simulink model "gm_transmitter"  (R2020b)
settings: Solver=FixedStepDiscrete  StartTime=0.0  StopTime=100000  RelTol=1e-3
undefined symbols (not defined in the file or in its folder): message
libraries: hdlmdlgenlib x98, dspsigops x53, hdlsllib x22, simulink x11, dspmlti4 x2, whdlio x1
(part 2 of 3)

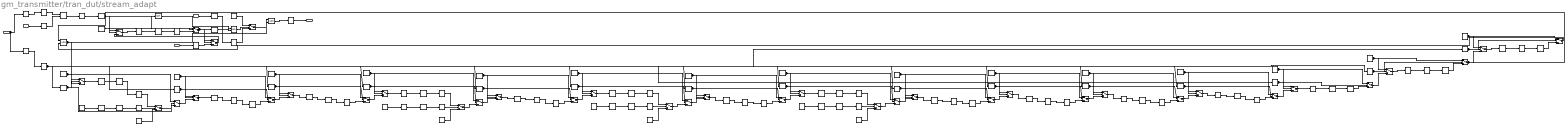
== system gm_transmitter/tran_dut/stream_adapt ==
  note: Padding unit
  input_bit : Inport  OutDataTypeStr=fixdt(0, 1, 0)  PortDimensions=1  SampleTime=2.06577425218972
  start : Inport  Port=2  OutDataTypeStr=boolean  PortDimensions=1  SampleTime=0.258221781523715
  valid : Inport  Port=3  OutDataTypeStr=boolean  PortDimensions=1  SampleTime=2.06577425218972
  end : Inport  Port=4  OutDataTypeStr=boolean  PortDimensions=1  SampleTime=0.258221781523715
  Compare To Constant : simulink/Logic and Bit Operations/Compare To Constant  relop=>=  const="fi(0,0,16,0,\"hex\",\"bd18\")"  OutDataTypeStr=boolean
  Compare To Constant1 : simulink/Logic and Bit Operations/Compare To Constant  relop===  const="fi(0,0,1,0,\"hex\",\"1\")"  OutDataTypeStr=boolean
  Constant : Constant  Value=0  OutDataTypeStr=fixdt(0, 1, 1000)  SampleTime=0.258221781523715
  Delay10_lowered : RateTransition  OutPortSampleTimeOpt=Multiple of input port sample time  OutPortSampleTimeMultiple=8
  Delay11_lowered : RateTransition  OutPortSampleTimeOpt=Multiple of input port sample time  OutPortSampleTimeMultiple=8
  Delay12_lowered : RateTransition  OutPortSampleTimeOpt=Multiple of input port sample time  OutPortSampleTimeMultiple=8
  Delay13_lowered : RateTransition  OutPortSampleTimeOpt=Multiple of input port sample time  OutPortSampleTimeMultiple=8
  Delay14_lowered : RateTransition  OutPortSampleTimeOpt=Multiple of input port sample time  OutPortSampleTimeMultiple=8
  Delay1_lowered : RateTransition  OutPortSampleTimeOpt=Multiple of input port sample time  OutPortSampleTimeMultiple=8
  Delay2_lowered : RateTransition  OutPortSampleTimeOpt=Multiple of input port sample time  OutPortSampleTimeMultiple=8
  Delay3_lowered : RateTransition  OutPortSampleTimeOpt=Multiple of input port sample time  OutPortSampleTimeMultiple=8
  Delay3_lowered_Initial_Val : Constant  OutDataTypeStr=boolean  SampleTime=0.258221781523715
  Delay3_lowered_ctrl_const : Constant  OutDataTypeStr=boolean  SampleTime=2.06577425218972
  Delay3_lowered_switch : Switch  Criteria=u2 ~= 0  Threshold=double(0)  OutDataTypeStr=boolean  SampleTime=0.258221781523715
  Delay4_lowered : RateTransition  OutPortSampleTimeOpt=Multiple of input port sample time  OutPortSampleTimeMultiple=8
  Delay5_lowered : RateTransition  OutPortSampleTimeOpt=Multiple of input port sample time  OutPortSampleTimeMultiple=8
  Delay5_lowered_Initial_Val : Constant  OutDataTypeStr=boolean  SampleTime=0.258221781523715
  Delay5_lowered_ctrl_const : Constant  OutDataTypeStr=boolean  SampleTime=2.06577425218972
  Delay5_lowered_switch : Switch  Criteria=u2 ~= 0  Threshold=double(0)  OutDataTypeStr=boolean  SampleTime=0.258221781523715
  Delay6_lowered : RateTransition  OutPortSampleTimeOpt=Multiple of input port sample time  OutPortSampleTimeMultiple=8
  Delay7_lowered : RateTransition  OutPortSampleTimeOpt=Multiple of input port sample time  OutPortSampleTimeMultiple=8
  Delay7_lowered_Initial_Val : Constant  OutDataTypeStr=boolean  SampleTime=0.258221781523715
  Delay7_lowered_ctrl_const : Constant  OutDataTypeStr=boolean  SampleTime=2.06577425218972
  Delay7_lowered_switch : Switch  Criteria=u2 ~= 0  Threshold=double(0)  OutDataTypeStr=boolean  SampleTime=0.258221781523715
  Delay8_lowered : RateTransition  OutPortSampleTimeOpt=Multiple of input port sample time  OutPortSampleTimeMultiple=8
  Delay9_lowered : RateTransition  OutPortSampleTimeOpt=Multiple of input port sample time  OutPortSampleTimeMultiple=8
  Delay_lowered : RateTransition  OutPortSampleTimeOpt=Multiple of input port sample time  OutPortSampleTimeMultiple=8
  Delay_lowered_Initial_Val : Constant  OutDataTypeStr=boolean  SampleTime=0.258221781523715
  Delay_lowered_ctrl_const : Constant  OutDataTypeStr=boolean  SampleTime=2.06577425218972
  Delay_lowered_switch : Switch  Criteria=u2 ~= 0  Threshold=double(0)  OutDataTypeStr=boolean  SampleTime=0.258221781523715
  From{,1..14} (15 alike) : hdlmdlgenlib/Buffer
      settings: SourceProductBaseCode=SL
  Goto : hdlmdlgenlib/Buffer
      settings: SourceProductBaseCode=SL
  Initial_Val{,1..7,9,11,13..14} (12 alike) : Constant  Value=0  OutDataTypeStr=boolean  SampleTime=0.258221781523715
  Initial_Val{8,10,12,15} (4 alike) : Constant  OutDataTypeStr=boolean  SampleTime=0.258221781523715
  Logical Operator : Logic  Operator=XOR  AllPortsSameDT=off  OutDataTypeStr=boolean  SampleTime=0.258221781523715
  Logical Operator1 : Logic  Operator=XOR  AllPortsSameDT=off  OutDataTypeStr=boolean  SampleTime=0.258221781523715
  Logical Operator2 : Logic  Operator=NOT  Inputs=1  AllPortsSameDT=off  OutDataTypeStr=boolean  SampleTime=0.258221781523715
  Logical Operator3 : Logic  AllPortsSameDT=off  OutDataTypeStr=boolean  SampleTime=0.258221781523715
  RateTransition : RateTransition  OutPortSampleTimeOpt=Multiple of input port sample time  OutPortSampleTimeMultiple=8
  Switch : Switch  Criteria=u2 ~= 0  Threshold=double(0)  OutDataTypeStr=boolean  SampleTime=0.258221781523715
  Switch1 : Switch  Criteria=u2 ~= 0  Threshold=double(0)  OutDataTypeStr=fixdt(0, 1, 0)  SampleTime=0.258221781523715
  crp_delay : Delay  DelayLength=double(1)  InitialCondition=0  SampleTime=0.258221781523715
  crp_out_delay{,1..15} (16 alike) : Delay  DelayLength=double(1)  InitialCondition=0  SampleTime=0.258221781523715
  delayMatch{,1..3,5,8..12} (10 alike) : Delay  DelayLength=double(1)  InitialCondition=0  SampleTime=2.06577425218972
  delayMatch4 : Delay  DelayLength=double(1)  InitialCondition=0  SampleTime=0.258221781523715
  delayMatch6 : Delay  DelayLength=double(8)  InitialCondition=0  SampleTime=0.258221781523715
  delayMatch7 : Delay  DelayLength=double(8)  InitialCondition=0  SampleTime=0.258221781523715
  ended_flag_lowered : RateTransition  OutPortSampleTimeOpt=Multiple of input port sample time  OutPortSampleTimeMultiple=8
  frame_counter : hdlsllib/Sources/HDL Counter  CountType=Count limited  CountInit=double(0)  CountStep=double(1)  CountMax=double(48408)  CountFromType=Initial value  CountFrom=double(0)  CountResetPort=on  CountLoadPort=off  CountEnbPort=on  CountDirPort=off  CountDataType=Unsigned  CountWordLen=16  CountFracLen=0  CountSampTime=2.06577425218972
  in10_repeat : dspsigops/Repeat  N=double(8)  RateOptions=Allow multirate processing  ic=0  mode=Unused parameter value
  in11_repeat : dspsigops/Repeat  N=double(8)  RateOptions=Allow multirate processing  ic=0  mode=Unused parameter value
  in12_repeat : dspsigops/Repeat  N=double(8)  RateOptions=Allow multirate processing  ic=0  mode=Unused parameter value
  in13_repeat : dspsigops/Repeat  N=double(8)  RateOptions=Allow multirate processing  ic=0  mode=Unused parameter value
  in14_repeat : dspsigops/Repeat  N=double(8)  RateOptions=Allow multirate processing  ic=0  mode=Unused parameter value
  in15_repeat : dspsigops/Repeat  N=double(8)  RateOptions=Allow multirate processing  ic=0  mode=Unused parameter value
  in16_repeat : dspsigops/Repeat  N=double(8)  RateOptions=Allow multirate processing  ic=0  mode=Unused parameter value
  in17_repeat : dspsigops/Repeat  N=double(8)  RateOptions=Allow multirate processing  ic=0  mode=Unused parameter value
  in18_repeat : dspsigops/Repeat  N=double(8)  RateOptions=Allow multirate processing  ic=0  mode=Unused parameter value
  in19_repeat : dspsigops/Repeat  N=double(8)  RateOptions=Allow multirate processing  ic=0  mode=Unused parameter value
  in20_repeat : dspsigops/Repeat  N=double(8)  RateOptions=Allow multirate processing  ic=0  mode=Unused parameter value
  in21_repeat : dspsigops/Repeat  N=double(8)  RateOptions=Allow multirate processing  ic=0  mode=Unused parameter value
  in22_repeat : dspsigops/Repeat  N=double(8)  RateOptions=Allow multirate processing  ic=0  mode=Unused parameter value
  in23_repeat : dspsigops/Repeat  N=double(8)  RateOptions=Allow multirate processing  ic=0  mode=Unused parameter value
  in2_repeat : dspsigops/Repeat  N=double(8)  RateOptions=Allow multirate processing  ic=0  mode=Unused parameter value
  in3_repeat : dspsigops/Repeat  N=double(8)  RateOptions=Allow multirate processing  ic=0  mode=Unused parameter value
  in4_repeat : dspsigops/Repeat  N=double(8)  RateOptions=Allow multirate processing  ic=0  mode=Unused parameter value
  in5_repeat : dspsigops/Repeat  N=double(8)  RateOptions=Allow multirate processing  ic=0  mode=Unused parameter value
  in6_repeat : dspsigops/Repeat  N=double(8)  RateOptions=Allow multirate processing  ic=0  mode=Unused parameter value
  in7_repeat : dspsigops/Repeat  N=double(8)  RateOptions=Allow multirate processing  ic=0  mode=Unused parameter value
  in8_repeat : dspsigops/Repeat  N=double(8)  RateOptions=Allow multirate processing  ic=0  mode=Unused parameter value
  in9_repeat : dspsigops/Repeat  N=double(8)  RateOptions=Allow multirate processing  ic=0  mode=Unused parameter value
  reset_in{,1..15} (16 alike) : Switch  Criteria=u2 ~= 0  Threshold=double(0)  OutDataTypeStr=boolean  SampleTime=0.258221781523715
  reset_out{,1..15} (16 alike) : Switch  Criteria=u2 ~= 0  Threshold=double(0)  OutDataTypeStr=boolean  SampleTime=0.258221781523715
  out : Outport  VectorParamsAs1DForOutWhenUnconnected=off
  wires:
  frame_counter/1 -> in23_repeat/1
  delayMatch11/1 -> in20_repeat/1
  delayMatch10/1 -> in16_repeat/1
  delayMatch9/1 -> in13_repeat/1
  delayMatch8/1 -> in10_repeat/1
  delayMatch12/1 -> in21_repeat/1
  delayMatch7/1 -> Goto/1
  delayMatch5/1 -> frame_counter/2
  delayMatch6/1 -> Switch/3
  crp_delay/1 -> RateTransition/1
  RateTransition/1 -> frame_counter/1
  input_bit/1 -> delayMatch12/1
  start/1 -> delayMatch7/1, crp_delay/1
  valid/1 -> delayMatch5/1
  end/1 -> delayMatch6/1
  delayMatch3/1 -> delayMatch8/1
  delayMatch2/1 -> delayMatch9/1
  delayMatch1/1 -> delayMatch10/1
  delayMatch/1 -> delayMatch11/1
  ended_flag_lowered/1 -> in22_repeat/1
  Delay_lowered/1 -> in19_repeat/1
  Delay1_lowered/1 -> in18_repeat/1
  Delay2_lowered/1 -> in17_repeat/1
  Delay3_lowered/1 -> in15_repeat/1
  Delay4_lowered/1 -> in14_repeat/1
  Delay5_lowered/1 -> in12_repeat/1
  Delay6_lowered/1 -> in11_repeat/1
  Delay7_lowered/1 -> in9_repeat/1
  Delay8_lowered/1 -> in8_repeat/1
  Delay9_lowered/1 -> in7_repeat/1
  Delay10_lowered/1 -> in6_repeat/1
  Delay11_lowered/1 -> in5_repeat/1
  Delay12_lowered/1 -> in4_repeat/1
  Delay13_lowered/1 -> in3_repeat/1
  Delay14_lowered/1 -> in2_repeat/1
  Delay_lowered_ctrl_const/1 -> delayMatch/1
  Delay3_lowered_ctrl_const/1 -> delayMatch1/1
  Delay5_lowered_ctrl_const/1 -> delayMatch2/1
  Delay7_lowered_ctrl_const/1 -> delayMatch3/1
  crp_out_delay/1 -> ended_flag_lowered/1
  crp_out_delay1/1 -> Delay_lowered/1
  crp_out_delay2/1 -> Delay1_lowered/1
  crp_out_delay3/1 -> Delay2_lowered/1
  crp_out_delay4/1 -> Delay3_lowered/1
  crp_out_delay5/1 -> Delay4_lowered/1
  crp_out_delay6/1 -> Delay5_lowered/1
  crp_out_delay7/1 -> Delay6_lowered/1
  crp_out_delay8/1 -> Delay7_lowered/1
  crp_out_delay9/1 -> Delay8_lowered/1
  crp_out_delay10/1 -> Delay9_lowered/1
  crp_out_delay11/1 -> Delay10_lowered/1
  crp_out_delay12/1 -> Delay11_lowered/1
  crp_out_delay13/1 -> Delay12_lowered/1
  crp_out_delay14/1 -> Delay13_lowered/1
  crp_out_delay15/1 -> Delay14_lowered/1
  in2_repeat/1 -> reset_out/3
  in3_repeat/1 -> reset_out1/3
  in4_repeat/1 -> reset_out2/3
  in5_repeat/1 -> reset_out3/3
  in6_repeat/1 -> reset_out4/3
  in7_repeat/1 -> reset_out5/3
  in8_repeat/1 -> reset_out6/3
  in9_repeat/1 -> Delay7_lowered_switch/1
  in10_repeat/1 -> Delay7_lowered_switch/2
  in11_repeat/1 -> reset_out8/3
  in12_repeat/1 -> Delay5_lowered_switch/1
  in13_repeat/1 -> Delay5_lowered_switch/2
  in14_repeat/1 -> reset_out10/3
  in15_repeat/1 -> Delay3_lowered_switch/1
  in16_repeat/1 -> Delay3_lowered_switch/2
  in17_repeat/1 -> reset_out12/3
  in18_repeat/1 -> reset_out13/3
  in19_repeat/1 -> Delay_lowered_switch/1
  in20_repeat/1 -> Delay_lowered_switch/2
  in21_repeat/1 -> Switch1/3
  in22_repeat/1 -> reset_out15/3
  in23_repeat/1 -> Compare To Constant/1
  delayMatch4/1 -> out/1
  Initial_Val/1 -> reset_out15/1, reset_in/1
  Switch/1 -> reset_in/3
  From9/1 -> reset_out5/2, reset_in6/2
  From8/1 -> reset_out6/2, reset_in7/2
  From7/1 -> reset_out7/2, reset_in8/2
  From6/1 -> reset_out8/2, reset_in9/2
  From5/1 -> reset_out9/2, reset_in10/2
  From4/1 -> reset_out10/2, reset_in11/2
  From3/1 -> reset_out11/2, reset_in12/2
  From2/1 -> reset_out12/2, reset_in13/2
  From13/1 -> reset_out1/2, reset_in2/2
  From12/1 -> reset_out2/2, reset_in3/2
  From11/1 -> reset_out3/2, reset_in4/2
  From10/1 -> reset_out4/2, reset_in5/2
  From1/1 -> reset_out13/2, reset_in14/2
  From/1 -> reset_out14/2, reset_in15/2
  Goto/1 -> From9/1, From8/1, From7/1, From6/1, From5/1, From4/1, From3/1, From2/1, From14/1, From13/1, From12/1, From11/1, From10/1, From1/1, From/1
  From14/1 -> reset_out/2, reset_in1/2
  reset_out/1 -> Logical Operator/2
  Initial_Val1/1 -> reset_out/1, reset_in1/1
  reset_out1/1 -> Logical Operator/1, reset_in1/3
  Initial_Val2/1 -> reset_out1/1, reset_in2/1
  reset_out2/1 -> reset_in2/3
  Initial_Val3/1 -> reset_out2/1, reset_in3/1
  reset_out3/1 -> reset_in3/3
  Initial_Val4/1 -> reset_out3/1, reset_in4/1
  reset_out4/1 -> reset_in4/3
  Initial_Val5/1 -> reset_out4/1, reset_in5/1
  reset_out5/1 -> reset_in5/3
  Initial_Val6/1 -> reset_out5/1, reset_in6/1
  reset_out6/1 -> reset_in6/3
  Initial_Val7/1 -> reset_out6/1, reset_in7/1
  Delay7_lowered_Initial_Val/1 -> Delay7_lowered_switch/3
  Delay7_lowered_switch/1 -> reset_out7/3
  reset_out7/1 -> reset_in7/3
  Initial_Val8/1 -> reset_out7/1, reset_in8/1
  reset_out8/1 -> reset_in8/3
  Initial_Val9/1 -> reset_out8/1, reset_in9/1
  Delay5_lowered_Initial_Val/1 -> Delay5_lowered_switch/3
  Delay5_lowered_switch/1 -> reset_out9/3
  reset_out9/1 -> reset_in9/3
  Initial_Val10/1 -> reset_out9/1, reset_in10/1
  reset_out10/1 -> reset_in10/3
  Initial_Val11/1 -> reset_out10/1, reset_in11/1
  Delay3_lowered_Initial_Val/1 -> Delay3_lowered_switch/3
  Delay3_lowered_switch/1 -> reset_out11/3
  reset_out11/1 -> reset_in11/3
  Initial_Val12/1 -> reset_out11/1, reset_in12/1
  reset_out12/1 -> reset_in12/3
  Initial_Val13/1 -> reset_out12/1, reset_in13/1
  reset_out13/1 -> reset_in13/3
  Initial_Val14/1 -> reset_out13/1, reset_in14/1
  Delay_lowered_Initial_Val/1 -> Delay_lowered_switch/3
  Delay_lowered_switch/1 -> reset_out14/3
  reset_out14/1 -> reset_in14/3
  Initial_Val15/1 -> reset_out14/1, reset_in15/1
  Logical Operator/1 -> Logical Operator1/1, reset_in15/3
  Constant/1 -> Switch1/1
  Switch1/1 -> Logical Operator1/2
  Logical Operator2/1 -> Logical Operator3/1
  Logical Operator3/1 -> Switch1/2
  Compare To Constant1/1 -> Logical Operator3/2
  reset_out15/1 -> Compare To Constant1/1, Switch/2, Switch/1
  Compare To Constant/1 -> Logical Operator2/1, reset_out15/2, reset_in/2
  reset_in/1 -> crp_out_delay/1
  reset_in15/1 -> crp_out_delay1/1
  reset_in14/1 -> crp_out_delay2/1
  reset_in13/1 -> crp_out_delay3/1
  reset_in12/1 -> crp_out_delay4/1
  reset_in11/1 -> crp_out_delay5/1
  reset_in10/1 -> crp_out_delay6/1
  reset_in9/1 -> crp_out_delay7/1
  reset_in8/1 -> crp_out_delay8/1
  reset_in7/1 -> crp_out_delay9/1
  reset_in6/1 -> crp_out_delay10/1
  reset_in5/1 -> crp_out_delay11/1
  reset_in4/1 -> crp_out_delay12/1
  reset_in3/1 -> crp_out_delay13/1
  reset_in2/1 -> crp_out_delay14/1
  reset_in1/1 -> crp_out_delay15/1
  Logical Operator1/1 -> delayMatch4/1

== system gm_transmitter/tran_dut/bch_encoder/output_mask ==
  bit_in : Inport  OutDataTypeStr=fixdt(0, 1, 0)  PortDimensions=1  SampleTime=0.258221781523715
  output_mask : MATLAB Function  TreatAsAtomicUnit=on
  mask : Outport  VectorParamsAs1DForOutWhenUnconnected=off
  wires:
  output_mask/1(mask) -> mask/1
  bit_in/1 -> output_mask/1(bit_in)

== system gm_transmitter/tran_dut/bch_encoder/p2s ==
  parallel_in : Inport  OutDataTypeStr=fixdt(0, 1, 0)  PortDimensions=[192]  SampleTime=2.06577425218972
  enable : Inport  Port=2  OutDataTypeStr=boolean  PortDimensions=1  SampleTime=2.06577425218972
  p2s : MATLAB Function  TreatAsAtomicUnit=on  mask{input_length=192}
  serial_out : Outport  VectorParamsAs1DForOutWhenUnconnected=off
  valid : Outport  Port=2
  wires:
  p2s/1(serial_out) -> serial_out/1
  p2s/2(valid) -> valid/1
  parallel_in/1 -> p2s/1(parallel_in)
  enable/1 -> p2s/2(enable)

== system gm_transmitter/tran_dut/bch_encoder/registers ==
  registers_in : Inport  OutDataTypeStr=fixdt(0, 1, 0)  PortDimensions=[192]  SampleTime=2.06577425218972
  registers : MATLAB Function  TreatAsAtomicUnit=on
  out : Outport  VectorParamsAs1DForOutWhenUnconnected=off
  registers_out : Outport  Port=2
  wires:
  registers/1(out) -> out/1
  registers/2(registers_out) -> registers_out/1
  registers_in/1 -> registers/1(registers_in)

== system gm_transmitter/tran_dut/bch_encoder/shift_and_xor ==
  input_bit : Inport  OutDataTypeStr=boolean  PortDimensions=1  SampleTime=0.258221781523715
  registers_in : Inport  Port=2  OutDataTypeStr=fixdt(0, 1, 0)  PortDimensions=[192]  SampleTime=0.258221781523715
  flag : Inport  Port=3  OutDataTypeStr=fixdt(0, 1, 0)  PortDimensions=[192]  SampleTime=0.258221781523715
  shift_and_xor : MATLAB Function  TreatAsAtomicUnit=on
  registers_out : Outport  VectorParamsAs1DForOutWhenUnconnected=off
  wires:
  shift_and_xor/1(registers_out) -> registers_out/1
  input_bit/1 -> shift_and_xor/1(input_bit)
  registers_in/1 -> shift_and_xor/2(registers_in)
  flag/1 -> shift_and_xor/3(flag)

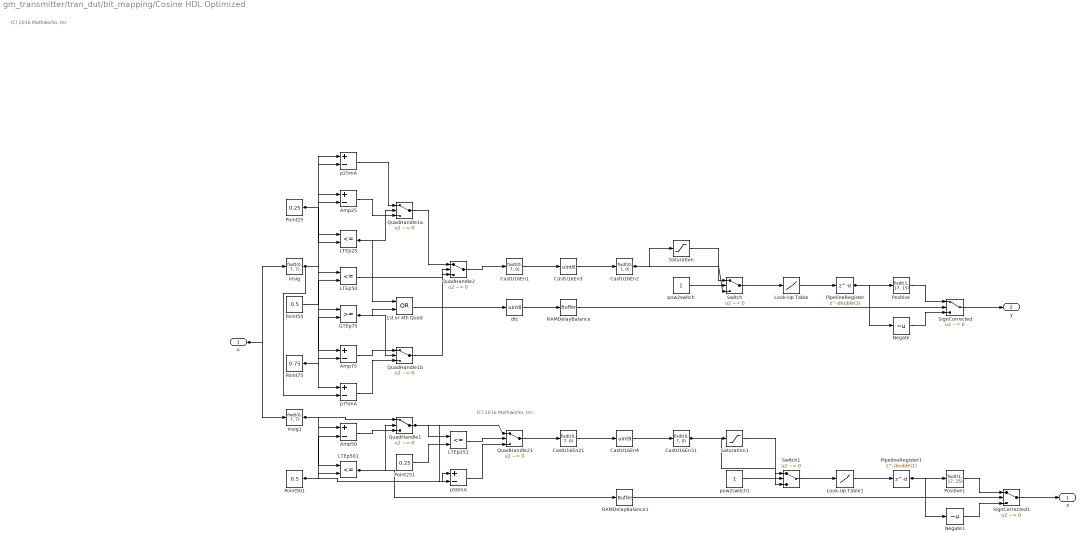
== system gm_transmitter/tran_dut/bit_mapping/Cosine HDL Optimized ==
  note: (C) 2016 Mathworks, Inc
  note: (C) 2016 Mathworks, Inc
  u : Inport  OutDataTypeStr=fixdt(1, 16, 14)  SampleTime=0.258221781523715
  1st or 4th Quad : Logic  Operator=OR  AllPortsSameDT=off  OutDataTypeStr=boolean  SampleTime=0.258221781523715
  Amp25 : Sum  Inputs=+-  AccumDataTypeStr=fixdt(1, 18, 17)  OutDataTypeStr=fixdt(1, 18, 17)  SampleTime=0.258221781523715
  Amp50 : Sum  Inputs=+-  AccumDataTypeStr=fixdt(1, 18, 17)  OutDataTypeStr=fixdt(1, 18, 17)  SampleTime=0.258221781523715
  Amp75 : Sum  Inputs=+-  AccumDataTypeStr=fixdt(1, 18, 17)  OutDataTypeStr=fixdt(1, 18, 17)  SampleTime=0.258221781523715
  CastU16En1 : DataTypeConversion  OutDataTypeStr=fixdt(0, 7, 0)  ConvertRealWorld=Stored Integer (SI)  SampleTime=0.258221781523715
  CastU16En2 : DataTypeConversion  OutDataTypeStr=fixdt(0, 7, 0)  ConvertRealWorld=Stored Integer (SI)  SampleTime=0.258221781523715  SaturateOnIntegerOverflow=on
  CastU16En21 : DataTypeConversion  OutDataTypeStr=fixdt(0, 7, 0)  ConvertRealWorld=Stored Integer (SI)  SampleTime=0.258221781523715
  CastU16En3 : DataTypeConversion  OutDataTypeStr=uint8  SampleTime=0.258221781523715
  CastU16En31 : DataTypeConversion  OutDataTypeStr=fixdt(0, 7, 0)  ConvertRealWorld=Stored Integer (SI)  SampleTime=0.258221781523715  SaturateOnIntegerOverflow=on
  CastU16En4 : DataTypeConversion  OutDataTypeStr=uint8  SampleTime=0.258221781523715
  GTEp75 : RelationalOperator  OutDataTypeStr=boolean  SampleTime=0.258221781523715  RndMeth=Nearest
  LTEp{25,50,251,501} (4 alike) : RelationalOperator  Operator=<=  OutDataTypeStr=boolean  SampleTime=0.258221781523715  RndMeth=Nearest
  Look-Up Table : Lookup_n-D  NumberOfTableDimensions=1  BreakpointsForDimension1="fi(\"numerictype\",numerictype(0,7,0),\"fimath\",fimath(\"RoundingMethod\", \"Floor\",\"OverflowAction\", \"Wrap\",\"ProductMode\",\"FullPrecision\",\"SumMode\",\"FullPrecision\"),\"Value\",\"[0 1 2 3 4 5 6 7 8 9 10 11 12 13 14 15 16 17 18 19 20 21 22 23 24 25 26 27 28 29 30 31]\")"  Table="reshape(fi(\"numerictype\",numerictype(1,17,15),\"fimath\",fimath(\"RoundingMethod\", \"Floor\",\"OverflowAction\", \"Wrap\",\"ProductMode\",\"FullPrecision\",\"SumMode\",\"FullPrecision\"),\"Value\",\"[0;0.0506591796875;0.101165771484375;0.15142822265625;0.2012939453125;0.250640869140625;0.29937744140625;0.3472900390625;0.39434814453125;0.440399169921875;0.48529052734375;0.528961181640625;0.571258544921875;0.612091064453125;0.6513671875;0.68896484375;0.72479248046875;0.758758544921875;0.790771484375;0.820770263671875;0.8486328125;0.874359130859375;0.897796630859375;0.9189453125;0.937744140625;0.954132080078125;0.96807861328125;0.979522705078125;0.98846435546875;0.994873046875;0.99871826171875;1]\"), [1  32])"  InterpMethod=Flat  ExtrapMethod=Clip  DiagnosticForOutOfRangeInput=Error  SampleTime=0.258221781523715  OutDataTypeStr=fixdt(1, 17, 15)  InputSameDT=on
  Look-Up Table1 : Lookup_n-D  NumberOfTableDimensions=1  BreakpointsForDimension1="fi(\"numerictype\",numerictype(0,7,0),\"fimath\",fimath(\"RoundingMethod\", \"Floor\",\"OverflowAction\", \"Wrap\",\"ProductMode\",\"FullPrecision\",\"SumMode\",\"FullPrecision\"),\"Value\",\"[0 1 2 3 4 5 6 7 8 9 10 11 12 13 14 15 16 17 18 19 20 21 22 23 24 25 26 27 28 29 30 31]\")"  Table="reshape(fi(\"numerictype\",numerictype(1,17,15),\"fimath\",fimath(\"RoundingMethod\", \"Floor\",\"OverflowAction\", \"Wrap\",\"ProductMode\",\"FullPrecision\",\"SumMode\",\"FullPrecision\"),\"Value\",\"[0;0.0506591796875;0.101165771484375;0.15142822265625;0.2012939453125;0.250640869140625;0.29937744140625;0.3472900390625;0.39434814453125;0.440399169921875;0.48529052734375;0.528961181640625;0.571258544921875;0.612091064453125;0.6513671875;0.68896484375;0.72479248046875;0.758758544921875;0.790771484375;0.820770263671875;0.8486328125;0.874359130859375;0.897796630859375;0.9189453125;0.937744140625;0.954132080078125;0.96807861328125;0.979522705078125;0.98846435546875;0.994873046875;0.99871826171875;1]\"), [1  32])"  InterpMethod=Flat  ExtrapMethod=Clip  DiagnosticForOutOfRangeInput=Error  SampleTime=0.258221781523715  OutDataTypeStr=fixdt(1, 17, 15)  InputSameDT=on
  Negate : UnaryMinus  SampleTime=0.258221781523715
  Negate1 : UnaryMinus  SampleTime=0.258221781523715
  PipelineRegister : Delay  DelayLength=double(1)  InitialCondition=0  SampleTime=0.258221781523715
  PipelineRegister1 : Delay  DelayLength=double(1)  InitialCondition=0  SampleTime=0.258221781523715
  Point25 : Constant  Value=0.25  OutDataTypeStr=fixdt(0, 17, 17)  SampleTime=0.258221781523715
  Point251 : Constant  Value=0.25  OutDataTypeStr=fixdt(0, 17, 17)  SampleTime=0.258221781523715
  Point50 : Constant  Value=0.5  OutDataTypeStr=fixdt(0, 17, 17)  SampleTime=0.258221781523715
  Point501 : Constant  Value=0.5  OutDataTypeStr=fixdt(0, 17, 17)  SampleTime=0.258221781523715
  Point75 : Constant  Value=0.75  OutDataTypeStr=fixdt(0, 17, 17)  SampleTime=0.258221781523715
  Positive : DataTypeConversion  OutDataTypeStr=fixdt(1, 17, 15)  SampleTime=0.258221781523715
  Positive1 : DataTypeConversion  OutDataTypeStr=fixdt(1, 17, 15)  SampleTime=0.258221781523715
  QuadHandle1 : Switch  Criteria=u2 ~= 0  Threshold=double(0)  OutDataTypeStr=fixdt(1, 18, 17)  SampleTime=0.258221781523715
  QuadHandle1a : Switch  Criteria=u2 ~= 0  Threshold=double(0)  OutDataTypeStr=fixdt(1, 18, 17)  SampleTime=0.258221781523715
  QuadHandle1b : Switch  Criteria=u2 ~= 0  Threshold=double(0)  OutDataTypeStr=fixdt(1, 18, 17)  SampleTime=0.258221781523715
  QuadHandle2 : Switch  Criteria=u2 ~= 0  Threshold=double(0)  OutDataTypeStr=fixdt(0, 7, 7)  SampleTime=0.258221781523715  SaturateOnIntegerOverflow=on
  QuadHandle21 : Switch  Criteria=u2 ~= 0  Threshold=double(0)  OutDataTypeStr=fixdt(0, 7, 7)  SampleTime=0.258221781523715
  RAMDelayBalance : hdlmdlgenlib/Buffer
      settings: SourceProductBaseCode=SL
  RAMDelayBalance1 : hdlmdlgenlib/Buffer
      settings: SourceProductBaseCode=SL
  Saturation : Saturate  UpperLimit="fi(0,0,7,0,\"hex\",\"1f\")"  LowerLimit="fi(0,0,7,0,\"hex\",\"00\")"  SampleTime=0.258221781523715  OutDataTypeStr=fixdt(0, 7, 0)
  Saturation1 : Saturate  UpperLimit="fi(0,0,7,0,\"hex\",\"1f\")"  LowerLimit="fi(0,0,7,0,\"hex\",\"00\")"  SampleTime=0.258221781523715  OutDataTypeStr=fixdt(0, 7, 0)
  SignCorrected : Switch  Criteria=u2 ~= 0  Threshold=double(0)  OutDataTypeStr=fixdt(1, 17, 15)  SampleTime=0.258221781523715
  SignCorrected1 : Switch  Criteria=u2 ~= 0  Threshold=double(0)  OutDataTypeStr=fixdt(1, 17, 15)  SampleTime=0.258221781523715
  Switch : Switch  Criteria=u2 ~= 0  Threshold=double(0)  OutDataTypeStr=fixdt(0, 7, 0)  SampleTime=0.258221781523715
  Switch1 : Switch  Criteria=u2 ~= 0  Threshold=double(0)  OutDataTypeStr=fixdt(0, 7, 0)  SampleTime=0.258221781523715
  dtc : DataTypeConversion  OutDataTypeStr=uint8  SampleTime=0.258221781523715
  insig : DataTypeConversion  OutDataTypeStr=fixdt(0, 7, 7)  SampleTime=0.258221781523715
  insig1 : DataTypeConversion  OutDataTypeStr=fixdt(0, 7, 7)  SampleTime=0.258221781523715
  p25mA : Sum  Inputs=+-  AccumDataTypeStr=fixdt(1, 18, 17)  OutDataTypeStr=fixdt(1, 18, 17)  SampleTime=0.258221781523715
  p50mA : Sum  Inputs=+-  AccumDataTypeStr=fixdt(1, 19, 17)  OutDataTypeStr=fixdt(1, 19, 17)  SampleTime=0.258221781523715
  p75mA : Sum  Inputs=+-  AccumDataTypeStr=fixdt(1, 18, 17)  OutDataTypeStr=fixdt(1, 18, 17)  SampleTime=0.258221781523715
  pow2switch : Constant  OutDataTypeStr=boolean  SampleTime=0.258221781523715
  pow2switch1 : Constant  OutDataTypeStr=boolean  SampleTime=0.258221781523715
  x : Outport
  y : Outport  Port=2
  wires:
  dtc/1 -> RAMDelayBalance/1
  Amp25/1 -> QuadHandle1a/3
  Amp75/1 -> QuadHandle1b/1
  CastU16En1/1 -> CastU16En3/1
  CastU16En2/1 -> Switch/3, Saturation/1
  CastU16En3/1 -> CastU16En2/1
  GTEp75/1 -> QuadHandle1b/2, 1st or 4th Quad/2
  LTEp25/1 -> QuadHandle1a/2, 1st or 4th Quad/1
  LTEp50/1 -> QuadHandle2/2
  PipelineRegister/1 -> Positive/1, Negate/1
  Negate/1 -> SignCorrected/3
  Point25/1 -> p25mA/1, LTEp25/2, Amp25/2
  Point50/1 -> LTEp50/2
  Point75/1 -> p75mA/1, GTEp75/2, Amp75/2
  Positive/1 -> SignCorrected/1
  QuadHandle1a/1 -> QuadHandle2/1
  QuadHandle1b/1 -> QuadHandle2/3
  QuadHandle2/1 -> CastU16En1/1
  Saturation/1 -> Switch/1
  SignCorrected/1 -> y/1
  Switch/1 -> Look-Up Table/1
  insig/1 -> p75mA/2, p25mA/2, LTEp50/1, LTEp25/1, GTEp75/1, Amp75/1, Amp25/1
  p25mA/1 -> QuadHandle1a/1
  p75mA/1 -> QuadHandle1b/3
  pow2switch/1 -> Switch/2
  Amp50/1 -> QuadHandle1/3
  CastU16En21/1 -> CastU16En4/1
  CastU16En31/1 -> Switch1/3, Saturation1/1
  CastU16En4/1 -> CastU16En31/1
  LTEp251/1 -> QuadHandle21/2
  LTEp501/1 -> QuadHandle1/2, RAMDelayBalance1/1
  PipelineRegister1/1 -> Positive1/1, Negate1/1
  Negate1/1 -> SignCorrected1/3
  Point251/1 -> LTEp251/2
  Point501/1 -> p50mA/1, LTEp501/2, Amp50/2
  Positive1/1 -> SignCorrected1/1
  QuadHandle1/1 -> p50mA/2, QuadHandle21/1, LTEp251/1
  QuadHandle21/1 -> CastU16En21/1
  Saturation1/1 -> Switch1/1
  SignCorrected1/1 -> x/1
  Switch1/1 -> Look-Up Table1/1
  insig1/1 -> QuadHandle1/1, LTEp501/1, Amp50/1
  p50mA/1 -> QuadHandle21/3
  pow2switch1/1 -> Switch1/2
  1st or 4th Quad/1 -> dtc/1
  RAMDelayBalance1/1 -> SignCorrected1/2
  RAMDelayBalance/1 -> SignCorrected/2
  u/1 -> insig1/1, insig/1
  Look-Up Table/1 -> PipelineRegister/1
  Look-Up Table1/1 -> PipelineRegister1/1

== system gm_transmitter/tran_dut/bit_mapping/angle_selector ==
  input : Inport  OutDataTypeStr=fixdt(0, 3, 0)  PortDimensions=1  SampleTime=0.258221781523715
  angle_selector : MATLAB Function  TreatAsAtomicUnit=on
  phase : Outport  VectorParamsAs1DForOutWhenUnconnected=off
  wires:
  angle_selector/1(phase) -> phase/1
  input/1 -> angle_selector/1(input)

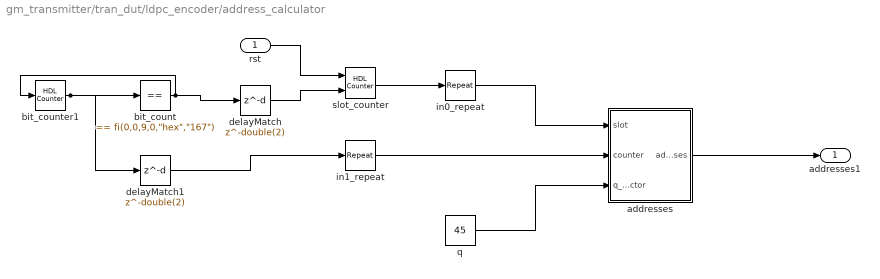
== system gm_transmitter/tran_dut/ldpc_encoder/address_calculator ==
  rst : Inport  OutDataTypeStr=boolean  PortDimensions=1  SampleTime=2.06577425218972
  addresses : Subsystem
  bit_count : simulink/Logic and Bit Operations/Compare To Constant  relop===  const="fi(0,0,9,0,\"hex\",\"167\")"  OutDataTypeStr=boolean
  bit_counter1 : hdlsllib/Sources/HDL Counter  CountType=Count limited  CountInit=double(0)  CountStep=double(1)  CountMax=double(359)  CountFromType=Initial value  CountFrom=double(0)  CountResetPort=on  CountLoadPort=off  CountEnbPort=off  CountDirPort=off  CountDataType=Unsigned  CountWordLen=9  CountFracLen=0  CountSampTime=2.06577425218972
  delayMatch : Delay  DelayLength=double(2)  InitialCondition=0  SampleTime=2.06577425218972
  delayMatch1 : Delay  DelayLength=double(2)  InitialCondition=0  SampleTime=2.06577425218972
  in0_repeat : dspsigops/Repeat  N=double(8)  RateOptions=Allow multirate processing  ic=0  mode=Unused parameter value
  in1_repeat : dspsigops/Repeat  N=double(8)  RateOptions=Allow multirate processing  ic=0  mode=Unused parameter value
  q : Constant  Value=45  OutDataTypeStr=uint8  SampleTime=0.258221781523715
  slot_counter : hdlsllib/Sources/HDL Counter  CountType=Count limited  CountInit=double(1)  CountStep=double(1)  CountMax=double(135)  CountFromType=Initial value  CountFrom=double(1)  CountResetPort=on  CountLoadPort=off  CountEnbPort=on  CountDirPort=off  CountDataType=Unsigned  CountWordLen=8  CountFracLen=0  CountSampTime=2.06577425218972
  addresses1 : Outport
  wires:
  delayMatch1/1 -> in1_repeat/1
  slot_counter/1 -> in0_repeat/1
  delayMatch/1 -> slot_counter/2
  addresses/1(addresses) -> addresses1/1
  rst/1 -> slot_counter/1
  bit_count/1 -> delayMatch/1, bit_counter1/1
  bit_counter1/1 -> delayMatch1/1, bit_count/1
  in0_repeat/1 -> addresses/1(slot)
  in1_repeat/1 -> addresses/2(counter)
  q/1 -> addresses/3(q_factor)

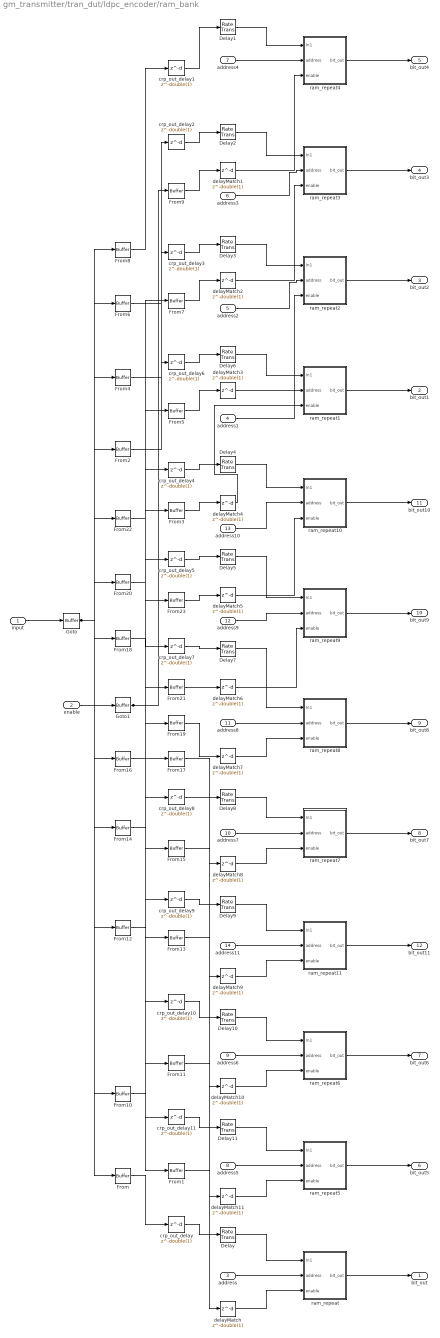
== system gm_transmitter/tran_dut/ldpc_encoder/ram_bank ==
  input : Inport  OutDataTypeStr=boolean  PortDimensions=1  SampleTime=0.258221781523715
  enable : Inport  Port=2  OutDataTypeStr=boolean  PortDimensions=1  SampleTime=2.06577425218972
  address : Inport  Port=3  OutDataTypeStr=fixdt(0, 14, 0)  PortDimensions=1  SampleTime=2.06577425218972
  address1 : Inport  Port=4  OutDataTypeStr=fixdt(0, 14, 0)  PortDimensions=1  SampleTime=2.06577425218972
  address2 : Inport  Port=5  OutDataTypeStr=fixdt(0, 14, 0)  PortDimensions=1  SampleTime=2.06577425218972
  address3 : Inport  Port=6  OutDataTypeStr=fixdt(0, 14, 0)  PortDimensions=1  SampleTime=2.06577425218972
  address4 : Inport  Port=7  OutDataTypeStr=fixdt(0, 14, 0)  PortDimensions=1  SampleTime=2.06577425218972
  address5 : Inport  Port=8  OutDataTypeStr=fixdt(0, 14, 0)  PortDimensions=1  SampleTime=2.06577425218972
  address6 : Inport  Port=9  OutDataTypeStr=fixdt(0, 14, 0)  PortDimensions=1  SampleTime=2.06577425218972
  address7 : Inport  Port=10  OutDataTypeStr=fixdt(0, 14, 0)  PortDimensions=1  SampleTime=2.06577425218972
  address8 : Inport  Port=11  OutDataTypeStr=fixdt(0, 14, 0)  PortDimensions=1  SampleTime=2.06577425218972
  address9 : Inport  Port=12  OutDataTypeStr=fixdt(0, 14, 0)  PortDimensions=1  SampleTime=2.06577425218972
  address10 : Inport  Port=13  OutDataTypeStr=fixdt(0, 14, 0)  PortDimensions=1  SampleTime=2.06577425218972
  address11 : Inport  Port=14  OutDataTypeStr=fixdt(0, 14, 0)  PortDimensions=1  SampleTime=2.06577425218972
  Delay{,1..11} (12 alike) : RateTransition  OutPortSampleTimeOpt=Multiple of input port sample time  OutPortSampleTimeMultiple=8
  From{,1..23} (24 alike) : hdlmdlgenlib/Buffer
      settings: SourceProductBaseCode=SL
  Goto : hdlmdlgenlib/Buffer
      settings: SourceProductBaseCode=SL
  Goto1 : hdlmdlgenlib/Buffer
      settings: SourceProductBaseCode=SL
  crp_out_delay{,1..11} (12 alike) : Delay  DelayLength=double(1)  InitialCondition=0  SampleTime=0.258221781523715
  delayMatch{,1..11} (12 alike) : Delay  DelayLength=double(1)  InitialCondition=0  SampleTime=2.06577425218972
  ram_repeat : Subsystem
  ram_repeat1 : Subsystem
  ram_repeat10 : Subsystem
  ram_repeat11 : Subsystem
  ram_repeat2 : Subsystem
  ram_repeat3 : Subsystem
  ram_repeat4 : Subsystem
  ram_repeat5 : Subsystem
  ram_repeat6 : Subsystem
  ram_repeat7 : Subsystem
  ram_repeat8 : Subsystem
  ram_repeat9 : Subsystem
  bit_out : Outport
  bit_out1 : Outport  Port=2
  bit_out2 : Outport  Port=3
  bit_out3 : Outport  Port=4
  bit_out4 : Outport  Port=5
  bit_out5 : Outport  Port=6
  bit_out6 : Outport  Port=7
  bit_out7 : Outport  Port=8
  bit_out8 : Outport  Port=9
  bit_out9 : Outport  Port=10
  bit_out10 : Outport  Port=11
  bit_out11 : Outport  Port=12
  wires:
  Delay/1 -> ram_repeat/1(In1)
  delayMatch/1 -> ram_repeat/3(enable)
  Delay11/1 -> ram_repeat5/1(In1)
  delayMatch11/1 -> ram_repeat5/3(enable)
  Delay10/1 -> ram_repeat6/1(In1)
  delayMatch10/1 -> ram_repeat6/3(enable)
  Delay9/1 -> ram_repeat11/1(In1)
  delayMatch9/1 -> ram_repeat11/3(enable)
  Delay8/1 -> ram_repeat7/1(In1)
  delayMatch8/1 -> ram_repeat7/3(enable)
  Delay7/1 -> ram_repeat8/1(In1)
  delayMatch7/1 -> ram_repeat8/3(enable)
  Delay6/1 -> ram_repeat1/1(In1)
  Delay5/1 -> ram_repeat9/1(In1)
  delayMatch6/1 -> ram_repeat9/3(enable)
  Delay4/1 -> ram_repeat10/1(In1)
  delayMatch5/1 -> ram_repeat10/3(enable)
  delayMatch4/1 -> ram_repeat1/3(enable)
  Delay3/1 -> ram_repeat2/1(In1)
  delayMatch3/1 -> ram_repeat2/3(enable)
  Delay2/1 -> ram_repeat3/1(In1)
  delayMatch2/1 -> ram_repeat3/3(enable)
  Delay1/1 -> ram_repeat4/1(In1)
  delayMatch1/1 -> ram_repeat4/3(enable)
  ram_repeat/1(bit_out) -> bit_out/1
  ram_repeat1/1(bit_out) -> bit_out1/1
  ram_repeat10/1(bit_out) -> bit_out10/1
  ram_repeat11/1(bit_out) -> bit_out11/1
  ram_repeat2/1(bit_out) -> bit_out2/1
  ram_repeat3/1(bit_out) -> bit_out3/1
  ram_repeat4/1(bit_out) -> bit_out4/1
  ram_repeat5/1(bit_out) -> bit_out5/1
  ram_repeat6/1(bit_out) -> bit_out6/1
  ram_repeat7/1(bit_out) -> bit_out7/1
  ram_repeat8/1(bit_out) -> bit_out8/1
  ram_repeat9/1(bit_out) -> bit_out9/1
  input/1 -> Goto/1
  enable/1 -> Goto1/1
  address/1 -> ram_repeat/2(address)
  address1/1 -> ram_repeat1/2(address)
  address2/1 -> ram_repeat2/2(address)
  address3/1 -> ram_repeat3/2(address)
  address4/1 -> ram_repeat4/2(address)
  address5/1 -> ram_repeat5/2(address)
  address6/1 -> ram_repeat6/2(address)
  address7/1 -> ram_repeat7/2(address)
  address8/1 -> ram_repeat8/2(address)
  address9/1 -> ram_repeat9/2(address)
  address10/1 -> ram_repeat10/2(address)
  address11/1 -> ram_repeat11/2(address)
  crp_out_delay/1 -> Delay/1
  crp_out_delay1/1 -> Delay1/1
  crp_out_delay2/1 -> Delay2/1
  crp_out_delay3/1 -> Delay3/1
  crp_out_delay4/1 -> Delay4/1
  crp_out_delay5/1 -> Delay5/1
  crp_out_delay6/1 -> Delay6/1
  crp_out_delay7/1 -> Delay7/1
  crp_out_delay8/1 -> Delay8/1
  crp_out_delay9/1 -> Delay9/1
  crp_out_delay10/1 -> Delay10/1
  crp_out_delay11/1 -> Delay11/1
  Goto/1 -> From8/1, From6/1, From4/1, From22/1, From20/1, From2/1, From18/1, From16/1, From14/1, From12/1, From10/1, From/1
  From/1 -> crp_out_delay/1
  From8/1 -> crp_out_delay1/1
  From6/1 -> crp_out_delay2/1
  From4/1 -> crp_out_delay3/1
  From22/1 -> crp_out_delay4/1
  From20/1 -> crp_out_delay5/1
  From2/1 -> crp_out_delay6/1
  From18/1 -> crp_out_delay7/1
  From16/1 -> crp_out_delay8/1
  From14/1 -> crp_out_delay9/1
  From12/1 -> crp_out_delay10/1
  From10/1 -> crp_out_delay11/1
  Goto1/1 -> From9/1, From7/1, From5/1, From3/1, From23/1, From21/1, From19/1, From17/1, From15/1, From13/1, From11/1, From1/1
  From1/1 -> delayMatch/1
  From9/1 -> delayMatch1/1
  From7/1 -> delayMatch2/1
  From5/1 -> delayMatch3/1
  From3/1 -> delayMatch4/1
  From23/1 -> delayMatch5/1
  From21/1 -> delayMatch6/1
  From19/1 -> delayMatch7/1
  From17/1 -> delayMatch8/1
  From15/1 -> delayMatch9/1
  From13/1 -> delayMatch10/1
  From11/1 -> delayMatch11/1

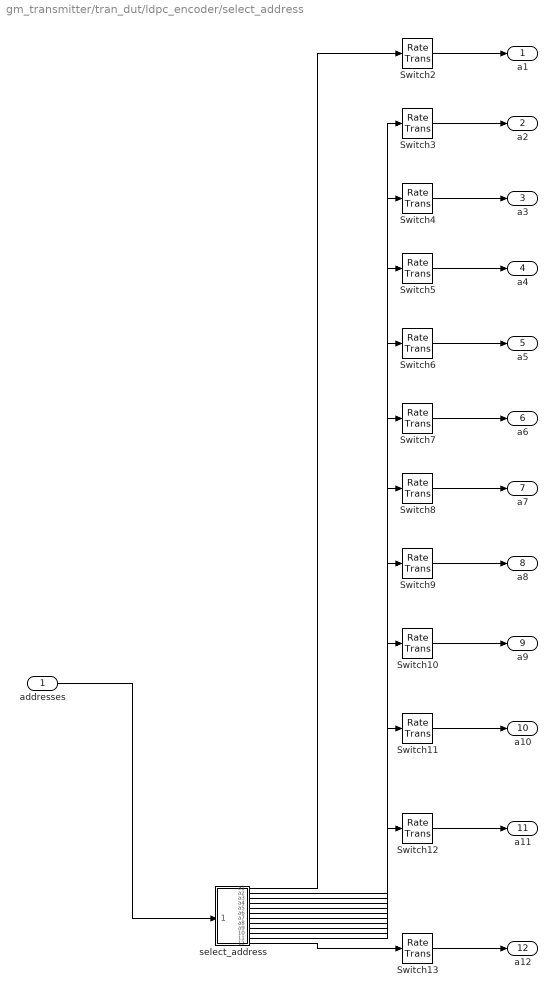
== system gm_transmitter/tran_dut/ldpc_encoder/select_address ==
  addresses : Inport  OutDataTypeStr=fixdt(0, 14, 0)  PortDimensions=[12]  SampleTime=0.258221781523715
  Switch{2..13} (12 alike) : RateTransition  OutPortSampleTimeOpt=Multiple of input port sample time  OutPortSampleTimeMultiple=8
  select_address : MATLAB Function  TreatAsAtomicUnit=on
  a1 : Outport  VectorParamsAs1DForOutWhenUnconnected=off
  a2 : Outport  Port=2
  a3 : Outport  Port=3
  a4 : Outport  Port=4
  a5 : Outport  Port=5
  a6 : Outport  Port=6
  a7 : Outport  Port=7
  a8 : Outport  Port=8
  a9 : Outport  Port=9
  a10 : Outport  Port=10
  a11 : Outport  Port=11
  a12 : Outport  Port=12
  wires:
  Switch2/1 -> a1/1
  Switch3/1 -> a2/1
  Switch4/1 -> a3/1
  Switch5/1 -> a4/1
  Switch6/1 -> a5/1
  Switch7/1 -> a6/1
  Switch8/1 -> a7/1
  Switch9/1 -> a8/1
  Switch10/1 -> a9/1
  Switch11/1 -> a10/1
  Switch12/1 -> a11/1
  Switch13/1 -> a12/1
  addresses/1 -> select_address/1(addresses)
  select_address/1(a1) -> Switch2/1
  select_address/2(a2) -> Switch3/1
  select_address/3(a3) -> Switch4/1
  select_address/4(a4) -> Switch5/1
  select_address/5(a5) -> Switch6/1
  select_address/6(a6) -> Switch7/1
  select_address/7(a7) -> Switch8/1
  select_address/8(a8) -> Switch9/1
  select_address/9(a9) -> Switch10/1
  select_address/10(a10) -> Switch11/1
  select_address/11(a11) -> Switch12/1
  select_address/12(a12) -> Switch13/1

== system gm_transmitter/tran_dut/ldpc_encoder/address_calculator/addresses ==
  slot : Inport  OutDataTypeStr=uint8  PortDimensions=1  SampleTime=0.258221781523715
  counter : Inport  Port=2  OutDataTypeStr=fixdt(0, 9, 0)  PortDimensions=1  SampleTime=0.258221781523715
  q_factor : Inport  Port=3  OutDataTypeStr=uint8  PortDimensions=1  SampleTime=0.258221781523715
  addresses1 : MATLAB Function  TreatAsAtomicUnit=on  mask{bit_addresses=uint16([[0 6385 7901 14611 13389 11200 3252 5243 2504 2722 821 7374]; [1 11359 2698 357 13824 12772 7244 6752 15310 852 2001 11417]; [2 7862 7977 6321 13612 12197 14449 15137 13860 1708 6399 13444]; [3 1560 11804 6975 13292 3646 3812 8772 7306 5795 14327 7866]; [4 7626 11407 14599 9689 1628 2113 10809 9283 1230 15241 4870]; [5 1610 5699 15876 9446 12515 1400 6303 5411 14181 13925 7358]; [6 4059 8836 3405 7853 7992 15336 5970 10368 10278 9675 4651]; [7 4441 3963 9153 2109 12683 7459 12030 12221 629 15212 406]; [8 6007 8411 5771 3497 543 14202 875 9186 6235 13908 3563]; [9 3232 6625 4795 546 9781 2071 7312 3399 7250 4932 12652]; [10 8820 10088 11090 7069 6585 13134 10158 7183 488 7455 9238]; [11 1903 10818 119 215 7558 11046 10615 11545 14784 7961 15619]; [12 3655 8736 4917 15874 5129 2134 15944 14768 7150 2692 1469]; [13 8316 3820 505 8923 6757 806 7957 4216 15589 13244 2622]; [14 14463 4852 15733 3041 11193 12860 13673 8152 6551 15108 8758]; [15 3149 11981 16200 16200 16200 16200 16200 16200 16200 16200 16200]; [16 13416 6906 16200 16200 16200 16200 16200 16200 16200 16200 16200]; [17 13098 13352 16200 16200 16200 16200 16200 16200 16200 16200 16200]; [18 2009 14460 16200 16200 16200 16200 16200 16200 16200 16200 16200]; [19 7207 4314 16200 16200 16200 16200 16200 16200 16200 16200 16200]; [20 3312 3945 16200 16200 16200 16200 16200 16200 16200 16200 16200]; [21 4418 6248 16200 16200 16200 16200 16200 16200 16200 16200 16200]; [22 2669 13975 16200 16200 16200 16200 16200 16200 16200 16200 16200]; [23 7571 9023 16200 16200 16200 16200 16200 16200 16200 16200 16200]; [24 14172 2967 16200 16200 16200 16200 16200 16200 16200 16200 16200]; [25 7271 7138 16200 16200 16200 16200 16200 16200 16200 16200 16200]; [26 6135 13670 16200 16200 16200 16200 16200 16200 16200 16200 16200]; [27 7490 14559 16200 16200 16200 16200 16200 16200 16200 16200 16200]; [28 8657 2466 16200 16200 16200 16200 16200 16200 16200 16200 16200]; [29 8599 12834 16200 16200 16200 16200 16200 16200 16200 16200 16200]; [30 3470 3152 16200 16200 16200 16200 16200 16200 16200 16200 16200]; [31 13917 4365 16200 16200 16200 16200 16200 16200 16200 16200 16200]; [32 6024 13730 16200 16200 16200 16200 16200 16200 16200 16200 16200]; [33 10973 14182 16200 16200 16200 16200 16200 16200 16200 16200 16200]; [34 2464 13167 16200 16200 16200 16200 16200 16200 16200 16200 16200]; [35 5281 15049 16200 16200 16200 16200 16200 16200 16200 16200 16200]; [36 1103 1849 16200 16200 16200 16200 16200 16200 16200 16200 16200]; [37 2058 1069 16200 16200 16200 16200 16200 16200 16200 16200 16200]; [38 9654 6095 16200 16200 16200 16200 16200 16200 16200 16200 16200]; [39 14311 7667 16200 16200 16200 16200 16200 16200 16200 16200 16200]; [40 15617 8146 16200 16200 16200 16200 16200 16200 16200 16200 16200]; [41 4588 11218 16200 16200 16200 16200 16200 16200 16200 16200 16200]; [42 13660 6243 16200 16200 16200 16200 16200 16200 16200 16200 16200]; [43 8578 7874 16200 16200 16200 16200 16200 16200 16200 16200 16200]; [44 11741 2686 16200 16200 16200 16200 16200 16200 16200 16200 16200]; [0 1022 1264 16200 16200 16200 16200 16200 16200 16200 16200 16200]; [1 12604 9965 16200 16200 16200 16200 16200 16200 16200 16200 16200]; [2 8217 2707 16200 16200 16200 16200 16200 16200 16200 16200 16200]; [3 3156 11793 16200 16200 16200 16200 16200 16200 16200 16200 16200]; [4 354 1514 16200 16200 16200 16200 16200 16200 16200 16200 16200]; [5 6978 14058 16200 16200 16200 16200 16200 16200 16200 16200 16200]; [6 7922 16079 16200 16200 16200 16200 16200 16200 16200 16200 16200]; [7 15087 12138 16200 16200 16200 16200 16200 16200 16200 16200 16200]; [8 5053 6470 16200 16200 16200 16200 16200 16200 16200 16200 16200]; [9 12687 14932 16200 16200 16200 16200 16200 16200 16200 16200 16200]; [10 15458 1763 16200 16200 16200 16200 16200 16200 16200 16200 16200]; [11 8121 1721 16200 16200 16200 16200 16200 16200 16200 16200 16200]; [12 12431 549 16200 16200 16200 16200 16200 16200 16200 16200 16200]; [13 4129 7091 16200 ...(+5412 chars)]]);, num_parity_bits=16200}
  addresses : Outport  VectorParamsAs1DForOutWhenUnconnected=off
  wires:
  addresses1/1(addresses) -> addresses/1
  slot/1 -> addresses1/1(slot)
  counter/1 -> addresses1/2(counter)
  q_factor/1 -> addresses1/3(q_factor)

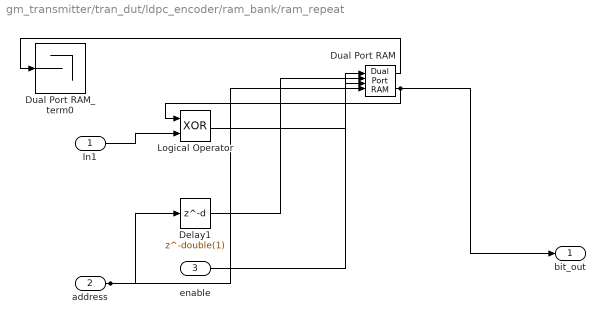
== system gm_transmitter/tran_dut/ldpc_encoder/ram_bank/ram_repeat ==
  In1 : Inport  OutDataTypeStr=boolean  PortDimensions=1  SampleTime=2.06577425218972
  address : Inport  Port=2  OutDataTypeStr=fixdt(0, 14, 0)  PortDimensions=1  SampleTime=2.06577425218972
  enable : Inport  Port=3  OutDataTypeStr=boolean  PortDimensions=1  SampleTime=2.06577425218972
  Delay1 : Delay  DelayLength=double(1)  InitialCondition=0  SampleTime=2.06577425218972
  Dual Port RAM : hdlsllib/HDL RAMs/Dual Port RAM  ram_size=14
      settings: SourceProductBaseCode=SL
  Dual Port RAM_term0 : Terminator
  Logical Operator : Logic  Operator=XOR  AllPortsSameDT=off  OutDataTypeStr=boolean  SampleTime=2.06577425218972
  bit_out : Outport
  wires:
  Delay1/1 -> Dual Port RAM/2
  Dual Port RAM/1 -> Dual Port RAM_term0/1
  Dual Port RAM/2 -> bit_out/1, Logical Operator/1
  In1/1 -> Logical Operator/2
  address/1 -> Delay1/1, Dual Port RAM/4
  enable/1 -> Dual Port RAM/3
  Logical Operator/1 -> Dual Port RAM/1

== system gm_transmitter/tran_dut/ldpc_encoder/ram_bank/ram_repeat1 ==
  In1 : Inport  OutDataTypeStr=boolean  PortDimensions=1  SampleTime=2.06577425218972
  address : Inport  Port=2  OutDataTypeStr=fixdt(0, 14, 0)  PortDimensions=1  SampleTime=2.06577425218972
  enable : Inport  Port=3  OutDataTypeStr=boolean  PortDimensions=1  SampleTime=2.06577425218972
  Delay1 : Delay  DelayLength=double(1)  InitialCondition=0  SampleTime=2.06577425218972
  Dual Port RAM : hdlsllib/HDL RAMs/Dual Port RAM  ram_size=14
      settings: SourceProductBaseCode=SL
  Dual Port RAM_term0 : Terminator
  Logical Operator : Logic  Operator=XOR  AllPortsSameDT=off  OutDataTypeStr=boolean  SampleTime=2.06577425218972
  bit_out : Outport
  wires:
  Delay1/1 -> Dual Port RAM/2
  Dual Port RAM/1 -> Dual Port RAM_term0/1
  Dual Port RAM/2 -> bit_out/1, Logical Operator/1
  In1/1 -> Logical Operator/2
  address/1 -> Delay1/1, Dual Port RAM/4
  enable/1 -> Dual Port RAM/3
  Logical Operator/1 -> Dual Port RAM/1
